simulink library "carnot"  (R2018b)
settings: Solver=VariableStepAuto  StartTime=0.0  StopTime=10.0  RelTol=1e-3
undefined symbols (not defined in the file or in its folder): A, A_earth, acol, Acol, ActPower1, ActPower2, ActPower3, Ad, Ad0, Ar, Au, Au0, Azimuth_Angle, B, Bd, Bd0, Br, Bu, Bu0, C, c1, c2, c3, c33, c4, c5, c6, CarnotCallbacks_Density, CarnotCallbacks_Enthalpy, CarnotCallbacks_Enthalpy2Temperature, CarnotCallbacks_Entropy, CarnotCallbacks_Evaporation_Enthalpy, CarnotCallbacks_GlobalMessageLevel, CarnotCallbacks_Grashof, CarnotCallbacks_Heat_Capacity, CarnotCallbacks_Kinematic_Viscosity, CarnotCallbacks_PMV_PPD, CarnotCallbacks_Prandtl, CarnotCallbacks_Saturation_Property, CarnotCallbacks_Saturation_Temperature, CarnotCallbacks_Saturation_Value_Water, CarnotCallbacks_Specific_Volume, CarnotCallbacks_Thermal_Conductivity, CarnotCallbacks_Vapour_Content, CarnotCallbacks_Vapour_Pressure, Cd, Cdl, Cr, Cu, Davies, Dd, DE_TRY2010_04_averageYear, delta_grd, density, DiameterLastPiece, dl, DPConstant, DPLinear, DPQuadratic, Dr ... (+59)
libraries: $bdroot x429, simulink x36, simulink_extras x12
(part 3 of 22)

== system carnot/Outputs ==
  AIV_selector : Subsystem  mask(AIV DATA){e1=on, e2=off, e3=off, e4=off, e5=off, e6=off, e7=off, e8=off, e9=off}
      mask prompts: e1 "Ts          : sensitive temperature, °C"; e2 "Tc          : convective/air temperature, °C"; e3 "Tr           : radiative temperature, °C"; e4 "x_H2O   : absolute water mass in air, kg/kg air"; e5 "x_CO2   : absolute CO2 mass in air, kg/kg air"; e6 "rho         : density of air, kg/m^3"; e7 "cp          : specific heat capacity of air, J/(kg*K)"; e8 "p            : absolute air pressure, N/m^2"; e9 "nair_out : air volume change indoors-outdoors, 1/h"
      mask help:
      | This block delivers a user specified vector with elements of the [AIV] vector.
      |
      | [AIV] : vector from NODE block
      | [AIV]s : output vector with user selected elements from [AIV]
      |
      | The sequence of elements in the output vector is identical to the sequence of selected check boxes counted from to the top to the bottom.
      mask init:
      | % concatenate elements of output "v":
      | v = [];
      | if (e1==1) v = [v 1]; end
      | if (e2==1) v = [v 2]; end
      | if (e3==1) v = [v 3]; end
      | if (e4==1) v = [v 4]; end
      | if (e5==1) v = [v 5]; end
      | if (e6==1) v = [v 6]; end
      | if (e7==1) v = [v 7]; end
      | if (e8==1) v = [v 8]; end
      | if (e9==1) v = [v 9]; end
      mask Help: web(fullfile(path_carnot('help'),'AIV_selector.html'),'-helpbrowser')
      mask Display:
      | plot ([0.8 0.9], [0.32 0.32])
      | plot ([0.8 0.85], [0.32 0.1])
      | plot ([0.9 0.85], [0.32 0.1])
      | plot ([0.827 0.827], [0 0.05])
      | plot ([0.827 0.87], [0.05 0.05])
      | plot ([0.87 0.87], [0 0.05])
      | plot ([0.827 0.87], [0 0])
  Display_THB1 : Subsystem  mask(display THB){t=on, m=off, p=off, id=off, mix=off, d=off}
      mask prompts: t "temperature [degree centigrade]"; m "massflow [kg/s]"; p "pressure [Pa]"; id "fluid ID (1 = water, 2 = air, 3 = cotton oil, 4 = water-glycol)"; mix "fluid mix"; d "diameter [m]"
      mask help: Displays the ticked values from one THB.
      mask init:
      | v=[];
      | if (t)
      |     v  = [2];
      | end
      | if (m)
      |     v= [v 3];
      | end
      | if (p)
      |     v = [v 4];
      | end
      | if (id)
      |     v = [v 5];
      | end
      | if (mix)
      |     v = [v 6];
      | end
      | if (d)
      |     v = [v 7];
      | end
      mask Help: web(fullfile(path_carnot('help'),'display_THB.html'),'-helpbrowser')
  Display_THB2 : Subsystem  mask(display THB){t=off, m=off, p=on, id=off, mix=off, d=off}
      mask prompts: t "temperature [degree centigrade]"; m "massflow [kg/s]"; p "pressure [Pa]"; id "fluid ID (1 = water, 2 = air, 3 = cotton oil, 4 = water-glycol)"; mix "fluid mix"; d "diameter [m]"
      mask help: Displays the ticked values from two THB.
      mask init:
      | v=[];
      | if (t)
      |     v  = [2];
      | end
      | if (m)
      |     v= [v 3];
      | end
      | if (p)
      |     v = [v 4];
      | end
      | if (id)
      |     v = [v 5];
      | end
      | if (mix)
      |     v = [v 6];
      | end
      | if (d)
      |     v = [v 7];
      | end
      mask Help: web(fullfile(path_carnot('help'),'display_THB.html'),'-helpbrowser')
  Display_THB3 : Subsystem  mask(display THB){t=off, m=off, p=on, id=off, mix=off, d=off}
      mask prompts: t "temperature [degree centigrade]"; m "massflow [kg/s]"; p "pressure [Pa]"; id "fluid ID (1 = water, 2 = air, 3 = cotton oil, 4 = water-glycol)"; mix "fluid mix"; d "diameter [m]"
      mask help: Displays the ticked values from four THB.
      mask init:
      | v=[];
      | if (t)
      |     v  = [2];
      | end
      | if (m)
      |     v= [v 3];
      | end
      | if (p)
      |     v = [v 4];
      | end
      | if (id)
      |     v = [v 5];
      | end
      | if (mix)
      |     v = [v 6];
      | end
      | if (d)
      |     v = [v 7];
      | end
      mask Help: web(fullfile(path_carnot('help'),'display_THB.html'),'-helpbrowser')
  Display_THB4 : Subsystem  mask(display THB){t=on, m=off, p=off, id=off, mix=off, d=off}
      mask prompts: t "temperature [degree centigrade]"; m "massflow [kg/s]"; p "pressure [Pa]"; id "fluid ID (1 = water, 2 = air, 3 = cotton oil, 4 = water-glycol)"; mix "fluid mix"; d "diameter [m]"
      mask help: Displays the ticked values from four THB
      mask init:
      | v=[];
      | if (t)
      |     v  = [2];
      | end
      | if (m)
      |     v= [v 3];
      | end
      | if (p)
      |     v = [v 4];
      | end
      | if (id)
      |     v = [v 5];
      | end
      | if (mix)
      |     v = [v 6];
      | end
      | if (d)
      |     v = [v 7];
      | end
      mask Help: web(fullfile(path_carnot('help'),'display_THB.html'),'-helpbrowser')
  Display_THB5 : Subsystem  mask(display THB){t=on, m=off, p=off, id=off, mix=off, d=off}
      mask prompts: t "temperature  [degree centigrade]"; m "massflow [kg/s]"; p "pressure [Pa]"; id "fluid ID (1 = water, 2 = air, 3 = cotton oil, 4 = water-glycol)"; mix "fluid mix"; d "diameter [m]"
      mask help: Displays the ticked values from six THB.
      mask init:
      | v=[];
      | if (t)
      |     v  = [2];
      | end
      | if (m)
      |     v= [v 3];
      | end
      | if (p)
      |     v = [v 4];
      | end
      | if (id)
      |     v = [v 5];
      | end
      | if (mix)
      |     v = [v 6];
      | end
      | if (d)
      |     v = [v 7];
      | end
      mask Help: web(fullfile(path_carnot('help'),'display_THB.html'),'-helpbrowser')
  Display_THB6 : Subsystem  mask(display THB){t=on, m=off, p=off, id=off, mix=off, d=off}
      mask prompts: t "temperature  [degree centigrade]"; m "massflow [kg/s]"; p "pressure [Pa]"; id "fluid ID (1 = water, 2 = air, 3 = cotton oil, 4 = water-glycol)"; mix "fluid mix"; d "diameter [m]"
      mask help: Displays the ticked values from six THB.
      mask init:
      | v=[];
      | if (t)
      |     v  = [2];
      | end
      | if (m)
      |     v= [v 3];
      | end
      | if (p)
      |     v = [v 4];
      | end
      | if (id)
      |     v = [v 5];
      | end
      | if (mix)
      |     v = [v 6];
      | end
      | if (d)
      |     v = [v 7];
      | end
      mask Help: web(fullfile(path_carnot('help'),'display_THB.html'),'-helpbrowser')
  PMV_PPD : Subsystem  LoadFcn=CarnotCallbacks_PMV_PPD('LoadFcn', gcb);  mask(PMV_PPD){DEBUGLEVEL=WARNINGLEVEL, MAXTOTALWARNINGS=inf, MAXCONSECUTIVEWARNINGS=inf, WRITETOFILE=0, FILENAME='messages.txt'}
      mask prompts: DEBUGLEVEL "Debug level"; MAXTOTALWARNINGS "maximum number of total warning"; MAXCONSECUTIVEWARNINGS "maximum number of consecutive warnings"; WRITETOFILE "write messages to file"; FILENAME "filename for messages"
      mask help:
      | This block calculates from it's inputs the thermal comfort according to PMV (pedicted mean vote) and PPD (predicted percentage of dissatisfied).
      | LoadPerPerson : metabolic rate of persons per surface in W/m² (typical 58.2 W/m²)
      | MechanicalLoad : effective mechanical power of a person in W/m²
      | ClothingIsolation : thermal resistance of the clothing in [m²/kW]; 1 clo = 0.155 W/m²
      | air temperature [°C]
      | radiation temperature [°C]
      | relative air velocity [m/s]
      | PartialPressureVapur : partial pressure of water [Pa]
      mask init:
      | %global debug level
      | [DEBUGLEVEL, MAXTOTALWARNINGS, MAXCONSECUTIVEWARNINGS, WRITETOFILE, FILENAME] = CarnotCallbacks_PMV_PPD('CheckDebugLevels', DEBUGLEVEL, MAXTOTALWARNINGS, MAXCONSECUTIVEWARNINGS, WRITETOFILE, FILENAME);
      mask Help: web(fullfile(path_carnot('help'),'PMV_PPD.html'),'-helpbrowser')
      mask TypeOptions DEBUGLEVEL: DEBUGLEVEL | INFOLEVEL | WARNINGLEVEL | ERRORLEVEL | FATALLEVEL | NOLEVEL
      mask Callback DEBUGLEVEL: CarnotCallbacks_PMV_PPD('MaskVisibilities');
      mask DialogControl ParameterTabVar0 Prompt: debugging air property calculations
  S_selector : Subsystem  mask(S_Selector){e1=on, e2=off, e3=off, e4=off, e5=off, e6=off, e7=off, e8=off, e9=off, e10=off, e11=off, e12=off, e13=off}
      mask prompts: e1 "Qdot_sol       : solar radition load, W"; e2 "Qdot_equip   : electric equipment load, W"; e3 "Qdot_light     : electric light load, W"; e4 "Qdot_pers     : person load, W"; e5 "Qdot_heat     : heating / cooling, W"; e6 "Qdot_air        : heating/cooling power of air change, W"; e7 "Qdot_c          : heat flow to convective node, W"; e8 "Qdot_r           : heat flow to radiative node, W"; e9 "mdot_air        : air mass flow, kg/s"; e10 "mdot_H2O    : water mass flow, kg/s"; e11 "mdot_CO2    : CO2 mass flow, kg/s"; e12 "Vdot_out2in  : air volume flow outdoors -> indoors, m^3/s"; e13 "Vdot_in2out  : air volume flow indoors -> outdoors, m^3/s"
      mask help:
      | This block delivers a user specified vector with elements of the [S] vector.
      |
      | [S] : vector from SOURCE or SINK block
      | [S]s : output vector with user selected elements from [S]
      |
      | The sequence of elements in the output vector is identical to the sequence of selected check boxes counted from to the top to the bottom.
      mask init:
      | % concatenate elements of output "v":
      | v = [];
      | if (e1==1) v = [v 1]; end
      | if (e2==1) v = [v 2]; end
      | if (e3==1) v = [v 3]; end
      | if (e4==1) v = [v 4]; end
      | if (e5==1) v = [v 5]; end
      | if (e6==1) v = [v 6]; end
      | if (e7==1) v = [v 7]; end
      | if (e8==1) v = [v 8]; end
      | if (e9==1) v = [v 9]; end
      | if (e10==1) v = [v 10]; end
      | if (e11==1) v = [v 11]; end
      | if (e12==1) v = [v 12]; end
      | if (e13==1) v = [v 13]; end
      mask Help: web(fullfile(path_carnot('help'),'S_selector.html'),'-helpbrowser')
      mask Display:
      | plot ([0.8 0.9], [0.32 0.32])
      | plot ([0.8 0.85], [0.32 0.1])
      | plot ([0.9 0.85], [0.32 0.1])
      | plot ([0.827 0.827], [0 0.05])
      | plot ([0.827 0.87], [0.05 0.05])
      | plot ([0.87 0.87], [0 0.05])
      | plot ([0.827 0.87], [0 0])
  Sensitive_Room_Temperature : Subsystem  mask(SENSITIVE TEMPERATURE){share_c=47}
      mask prompts: share_c "SHARE of convective sensitivity, [0,100%]:"
      mask help:
      | This block merges the convective and radiative zone node temperature to the SENSITIVE ZONE TEMPERATURE (weighted arithmetic average of both components).
      | [T] = [Tc; Tr]:  temperature vector of node, °C
      | Ts:              sensitive zone temperature, °C
      mask init:
      | blockname = gcb;
      | 
      | if (length(share_c)~=1) error(['PARAMETERS block "' blockname ': "SHARE of ..." must have only 1 entry !']); end;
      | if (share_c<0) | (share_c>100) error(['PARAMETERS block "' blockname '" : "SHARE of ..." must be within [0, 100%] !']); end;
      | share_c = share_c/100;
      mask Help: web(fullfile(path_carnot('help'),'Sensitive_room_temperature.html'),'-helpbrowser')
  THV_select : Subsystem  mask(select from THV){f=off, t=on, m=off, p=off, id=off, mix=off, d=off, dpcon=off, dplin=off, dpqua=off}
      mask prompts: f "flow identifier"; t "temperature [degree centigrade]"; m "massflow [kg/s]"; p "pressure [Pa]"; id "fluid ID (1 = water, 2 = air, 3 = cotton oil, 4 = water-glycol)"; mix "fluid mix"; d "diameter [m]"; dpcon "constant press. drop"; dplin "linear pressure drop"; dpqua "quadratic pressure drop"
      mask help: Selects the ticked values from the thermo hydraulic vector.
      mask init:
      | v=[];
      | if (f)
      |     v  = [1];
      | end
      | if (t)
      |     v  = [v 2];
      | end
      | if (m)
      |     v= [v 3];
      | end
      | if (p)
      |     v = [v 4];
      | end
      | if (id)
      |     v = [v 5];
      | end
      | if (mix)
      |     v = [v 6];
      | end
      | if (d)
      |     v = [v 7];
      | end
      | if (dpcon)
      |     v = [v 8];
      | end
      | if (dplin)
      |     v = [v 9];
      | end
      | if (dpqua)
      |     v = [v 10];
      | end
      mask Help: eval('man(''THV_select'')')
  display_weather : Subsystem  mask(Select weather data){pos=off, sun_beam=off, sun_dfu=off, rad=on, ta=off, ts=off, pre=off, rh=off, ci=off, p=off, ws=off, wd=off, col=off}
      mask prompts: pos "sunposition [zenith azimuth incidence] angles [degree]"; sun_beam "solar beam radiation on a normal surface [W/m²]"; sun_dfu "solar diffuse radiation on a horizontal surface [W/m²]"; rad "solar radiation on the surface [direct diffuse] [W/m²]"; ta "ambient temperature [degree centigrade]"; ts "sky temperature [degree centigrade]"; pre "precipitation [m/s]"; rh "relative humidity [percent]"; ci "cloud index [0=no cloud 1= covered]"; p "pressure [Pa]"; ws "wind speed [m/s]"; wd "wind direction (0°=north 270°=east) [degree]"; col "collector [incidence parallel_incidence perpendicular] [degree]"
      mask help: Selects the ticked weather data from the input weather data vector.
      mask init:
      | v=[];
      | if (pos)
      |     v  = [2 3 14];
      | end
      | if (sun_beam)
      |     v= [v 4];
      | end
      | if (sun_dfu)
      |     v= [v 5];
      | end
      | if (rad)
      |     v= [v 17 18];
      | end
      | if (ta)
      |     v = [v 6];
      | end
      | if (ts)
      |     v = [v 7];
      | end
      | if (rh)
      |     v = [v 8];
      | end
      | if (pre)
      |     v = [v 9];
      | end
      | if (ci)
      |     v = [v 10];
      | end
      | if (p)
      |     v = [v 11];
      | end
      | if (ws)
      |     v = [v 12];
      | end
      | if (wd)
      |     v = [v 13];
      | end
      | if (col)
      |     v = [v 14 15 16];
      | end
      mask Help: web(fullfile(path_carnot('help'),'display_weather.html'),'-helpbrowser')
  printer : S-Function  FunctionName=printer  SFunctionDeploymentMode=off  EnableBusSupport=off  mask(printer){}
      mask help: Print the input to the MATLAB command window during iterations of SIMULINK
      mask Help: web(fullfile(path_carnot('help'),'printer.html'),'-helpbrowser')

== system carnot/Source ==
  Boiler : Subsystem
      mask Display: plot(-20,0,120,100,[10,90,90,10,10],[10,10,20,20,10],[80,80,20,20],[20,90,90,20],[20,70,70,20],[24,24,30,30],[32,30,28],[30,40,30],[43,40,38],[30,40,30],[53,50,47],[30,40,30],[63,60,57],[30,40,30],[35,32,30,29,31,36,39,40,37,35],[75,69,65,58,50,49,53,59,68,75],[57,54,51,51,53,58,62,62,59,57],[76,71,67,58,49,48,54,60,69,76])
  Chiller : Subsystem
      mask Display: plot(20,20,80,100,(100-[30,46,36,46,36,46,30]),[40,40,50,60,70,80,80],(100-[70,54,64,54,64,54,64,54,64,54,70]),[40,40,44,50,55,60,65,70,75,80,80],[56,45],[95,95],[51,51],[82,95])
  Cogeneration : Subsystem
      mask Display: plot(0.1, 0, 0.9, 1,([0,8,20,30,42,50,50,42,30,20,8,0,0]+20)/140, [60,74,80,80,74,60,40,27,20,20,27,40,60]/100,([40,40,25,10,10]+20)/140,[40,60,50,60,40]/100,[60,50]/100,[50,50]/100,[60,80,80,60,60]/100, [30,30,70,70,30]/100,([90,97,97,90,80,75,75,80,90,97]+12)/140, [50,50,40,35,35,40,60,65,65,60]/100)
  Electric_Generator : Subsystem
      mask Display: plot(0,0,100,100,[40,20],[50,50],[40,40],[30,70],[50,50],[-0,100],[70,50],[50,50])
  Energy : Subsystem
      mask Display: plot(0,-0.1,0.8,1,[90,67,84,63,80,60,70,90,80,80,70,20,10,10,20,60]/120,[70,87,64,83,60,80,90,70,60,10,0,0,10,70,80,80]/100,[30,60,60,40,40,50,50,40,40,30,30]/120,[60,60,50,50,40,40,30,30,10,10,60]/100)
  Heat_Exchanger : Subsystem
      mask Display: plot(0,0,100,100,[70,30,30,70,70,30],[90,10,90,90,10,10])
  Heat_Pump : Subsystem
      mask Display: plot(20,20,80,100,[30,46,36,46,36,46,30],[40,40,50,60,70,80,80],[70,54,64,54,64,54,64,54,64,54,70],[40,40,44,50,55,60,65,70,75,80,80],[56,45],[95,95],[51,51],[82,95])
  Simple : Subsystem
      mask Display: plot(0,0,100,100,[30,40,60,70,70,30,30],[50,44,44,50,10,10,50],[50,50],[44,57],[50,46,44,46,50,54,56,54,50],[93,85,70,54,48,54,70,85,93])
  Solar_Thermal : Subsystem
      mask Display: plot(0,0,100,100,[0,10,16,19,20],[80,81,84,90,100],[7,10],[79,60],[17,30],[84,70],[21,40],[94,90],[30,90,100,40,30],[10,70,60,-0,10],[90,90,40,33],[70,60,10,13],[89,39],[61,12])
  Ventilation : Subsystem
      mask Display:
      | plot([0.2 0.35], [0.8 0.7])
      | plot([0.35 0.65], [0.7 0.7])
      | plot([0.65 0.8], [0.7 0.8])
      | plot([0.65 0.8], [0.76 0.8])
      | plot([0.7 0.8], [0.65 0.8])
      | plot([0.2 0.35], [0.2 0.3])
      | plot([0.35 0.65], [0.3 0.3])
      | plot([0.65 0.8], [0.3 0.2])
      | plot([0.2 0.25], [0.2 0.32])
      | plot([0.2 0.35], [0.2 0.23])
      | plot ([0.45 0.45], [0 1])
      | plot ([0.55 0.55], [0 1])
      | plot ([0.45 0.55], [0.2 0.2])
      | plot ([0.45 0.55], [0.8 0.8])
      | plot ([0.45 0.55], [0 0.2])
      | plot ([0.45 0.55], [0.8 1])

== system carnot/Storage ==
  Electric : Subsystem
      mask Display: plot(0,-10,100,100,[70,70,60,40,30,30,40,60,70,60,40,30],[80,10,-0,-0,10,80,70,70,80,90,90,80],[44,47,54,57,54,47,44],[80,76,76,80,84,84,80])
  Thermal : Subsystem
      mask Display: plot(30,40,60,90,[36,36,40,50,54,54,50,40,36],[90,50,45,45,50,90,93,93,90],[36,51,40,51,36],[74,74,79,85,85],[36,51,44,51,36],[54,54,56,58,58])

== system carnot/Toolbox ==
  Average : Subsystem  mask{time_intervall=3600, offset_flag=off, enable_flag=off}
      mask prompts: time_intervall "Delta_t in s"; offset_flag "start calculating every full hour"; enable_flag "only calculate when enabled"
      mask help:
      | This block calculates the average of each input vector during a specified time Delta_t. During this time interval the output is held.
      | The output time is the time of the last average calculation. Every time the average is calculated again, a signal pulse of 1 is put out.
      | When the full hour flag is set, the calculation of the average is started every full hour once again.
      | When the enable flag is set, the functions calculates only while the enable signal is 1. When it is 0, the function repeats putting out the last output.
      mask init:
      | if time_intervall==0
      |     delta_t = 1;
      | else
      |     delta_t = time_intervall;
      | end
      mask Help: web(fullfile(path_carnot('help'),'Average.html'),'-helpbrowser')
  Count_Working_Time : S-Function  FunctionName=countcycles  SFunctionDeploymentMode=off  EnableBusSupport=off  mask(count working time){}
      mask help: This block counts the number of on cycles and the working time (time when input is above zero).
      mask Help: web(fullfile(path_carnot('help'),'Count_Working_Time.html'),'-helpbrowser')
      mask Display:
      | port_label('input', 1, 'Input')
      | port_label('output', 1, 'flank')
      | port_label('output', 2, 'cycles')
      | port_label('output', 3, 'actual worktime')
      | port_label('output', 4, 'total worktime')
  Date2Sec : S-Function  FunctionName=date2sec_s  SFunctionDeploymentMode=off  EnableBusSupport=off
      mask help:
      | This function calculates for a given date the sum of seconds in the year.
      | The input Year is a dummy argument.
      | 0 s is january, 1st at 0:00:00.
      |
      | INPUT VECTOR:
      | date [year month day hour minute second]
      |
      | OUTPUT VECTOR:
      | date [s]
  Economy_Ecology : Subsystem  mask(economy_ecology){}
      mask help: Calculates massflow, costs, exhaust gas etc.
      mask Help: web(fullfile(path_carnot('help'),'economy_ecology.html'),'-helpbrowser')
  GlobalMessageLevel : Subsystem  LoadFcn=CarnotCallbacks_GlobalMessageLevel('LoadFcn');  mask(Global Message Level){GLOBALLOCAL=local, DEBUGLEVEL=DEBUG, MAXTOTALWARNINGS=inf, MAXCONSECUTIVEWARNINGS=inf, WRITETOFILE=0, FILENAME='error.txt'}
      mask prompts: GLOBALLOCAL "message settings"; DEBUGLEVEL "message level"; MAXTOTALWARNINGS "maximum total number of warnings"; MAXCONSECUTIVEWARNINGS "maxmum consecutive warnings"; WRITETOFILE "write messages to file"
      mask help:
      | This block sets the message level of the complete model. Error messages and warnings are generated for example by the material properties functions (density, ...), see library Basic/Material_Properties for the blocks.
      | local - settings are defined by each block individually
      | global - settings are defined by this GlobalMessageLevel block
      | Copy this block once in the model if you want to use a global handling of Carnot error messages.
      mask init:
      | CarnotCallbacks_GlobalMessageLevel('SetData');
      mask TypeOptions GLOBALLOCAL: global | local
      mask Callback GLOBALLOCAL: CarnotCallbacks_GlobalMessageLevel('MaskCallback');
      mask TypeOptions DEBUGLEVEL: DEBUGLEVEL | INFOLEVEL | WARNINGLEVEL | ERRORLEVEL | FATALLEVEL | NOLEVEL
      mask Display:
      | fprintf(get_param(gcb, 'GLOBALLOCAL'));
      | fprintf(['\n\n', get_param(gcb, 'DEBUGLEVEL')]);
  ModelDoc : Subsystem  mask(ModelDoc){}
      mask init:
      | % modelname=bdroot;
      | % filename=[modelname '_params.txt'];
      | % fid = fopen(filename, 'w');
      | % line='______________________________________________________';
      | % ttt=SearchWriteParams(modelname,fid);
      | % fclose(fid);
      | 
      | ok = CarnotCallbacks_ModelDoc;
      settings: OpenFcn=|
      | if  ~BlockIsInCarnotLibrary
      |     modelname=get_param(0,'CurrentSystem');
      |     filename=[modelname '_params.txt'];
      |     open(filename);
      | end
      mask Display: disp('Model Description\n Update Model <Ctrl>D \n before double-clicking');
  RealDate : Subsystem  mask{form=second}
      mask prompts: form "Selector"
      mask help:
      | This functions puts out the system time and date:
      | Year - current year
      | Month - current month
      | Day - current day in the month (date)
      | Hour -  current hour (time)
      | Minute - current minute (of the time)
      | Second - current second (of the time)
      mask Help: web(fullfile(path_carnot('help'),'RealDate.html'),'-helpbrowser')
      mask TypeOptions form: year | month | day | hour | minute | second
  RealTime : Subsystem
      mask help:
      | This functions puts out the system time in seconds.
      | Output 0 s means January, 1st 0:00
      mask Help: web(fullfile(path_carnot('help'),'RealTime.html'),'-helpbrowser')
  RealTimePulse : Subsystem  mask{typ=rising, time=3}
      mask prompts: typ "type"; time "time interval [s]"
      mask help:
      | This functions creates a signal pulse, whenever the input pulse is
      | changing as specified. The duration of the pulse is depending on the system time, not the simulation time.
      |
      | INPUT VECTOR:
      |   in : signal to start pulse [0,1]
      |
      | OUTPUT VECTOR:
      |  out : new pulse [0,1]
      mask Help: web(fullfile(path_carnot('help'),'RealTimePulse.html'),'-helpbrowser')
      mask TypeOptions typ: rising | falling | either
  Sec2Date : S-Function  FunctionName=sec2date_s  SFunctionDeploymentMode=off  EnableBusSupport=off
      mask help:
      | This functions calculates from a given number of seconds the date.
      |
      | INPUT VECTOR:
      | - time [s]
      |
      | OUTPUT VECTOR:
      | - date [month day hour minute second]
  SumTime : S-Function  FunctionName=sumtime_s  SFunctionDeploymentMode=off  EnableBusSupport=off
      mask help:
      | This function calcultes for a given date the sum of seconds, minutes, ... in the year.
      |
      | INPUT VECTOR:
      | date [year month day hour minute second]
      |
      | OUTPUT VECTOR:
      | sum of |year month day hour minute second]
      mask Help: web(fullfile(path_carnot('help'),'SumTime_mdl.html'),'-helpbrowser')
      mask Display: plot(0,0,70,60,[40 20 35 20 40],[50 50 30 10 10],[50 50 45 55 50  50 52 54],[45 35 35 35 35 20 17 15]);
  SystemPulse : Subsystem  mask(system pulse){enable_flag=on, datecheck=off, date=[2 10 10 36 15], period=5, pulsewidth=2}
      mask prompts: enable_flag "Wait for enabling pulse"; datecheck "Wait for start date"; date "start date [month day hour minute second]"; period "period [s]"; pulsewidth "pulse width [s]"
      mask help:
      | This block generates a discrete pulse of 0 and 1, but this pulse depends on the system time, not the simulation time.
      | If the date flag is set, the function starts pulsing only when the system date reaches the specified date. Otherwise the output is 0.
      | If the enable flag is set, the function waits, until the enabling pulse once rise from 0 to 1. Afterwards the pulsing is started. Before pulsing the output will be 0.
      mask Help: web(fullfile(path_carnot('help'),'SystemPulse.html'),'-helpbrowser')
  THB2THV : Subsystem  InitFcn=load('THB.mat');  mask(THB2THV){}
      mask help: This block converts the Thermo-Hydraulic-Bus to the old Thermo-Hydraulic-Vector.
      mask Help: web(fullfile(path_carnot('help'),'THB2THV.html'),'-helpbrowser')
  THBMemory : Subsystem  InitFcn=load('THB.mat');  mask(THB Memory){ID=20001, T=20, mdot=0, p=1e5, FluidType=1, FluidMix=0, d=0.01, c=0, l=0, q=0, LH=1000, H=0, Annotation_ID=off, Annotation_T=off, Annotation_mdot=off, Annotation_p=off, Annotation_FluidType=off, Annotation_FluidMix=off, Annotation_d=off, Annotation_c=off, Annotation_l=off, Annotation_q=off, Annotation_LH=off, Annotation_H=off}
      mask prompts: ID "Fluid ID [1]"; T "Temperature [°C]"; mdot "Mass flow rate [kg/s]"; p "Pressure [Pa]"; FluidType "Fluid type [enum]"; FluidMix "Fluid mix [1]"; d "Diameter of the last piece [m]"; c "Constant pressure drop coefficient [Pa]"; l "Linear pressure drop coefficient [Pa/(kg/s)]"; q "Quadratic pressure drop coefficient [Pa/(kg/s)²]"; LH "Hydraulic inductance [1/m]"; H "Geodetic height [m]"; Annotation_ID "Fluid ID as annotation"; Annotation_T "Temperature as annoation"; Annotation_mdot "Mass flow rate as annoation"; Annotation_p "Pressure as annotation"; Annotation_FluidType "Fluid type as annotation"; Annotation_FluidMix "Fluid mix as annotation"; Annotation_d "Diameter of the last piece as annotation"; Annotation_c "Constant pressure drop coefficient as annotation"; Annotation_l "Linear pressure drop coefficient as annotation"; Annotation_q "Quadratic pressure drop coefficient as annotation"; Annotation_LH "Hydraulic inductance as annotation"; Annotation_H "Geodetic height as annotation"
      mask help: This is a memory block for a complete THB.
      mask init:
      | %annotations    
      | MaskValues=get_param(gcb,'MaskValues');
      | AnnotationString='';
      | if strcmp(MaskValues{13},'on') %ID
      |     if ~isempty(AnnotationString)
      |         AnnotationString=[AnnotationString,sprintf('\n')];
      |     end
      |     AnnotationString=[AnnotationString,'ID ',MaskValues{1}];
      | end
      |     
      | if strcmp(MaskValues{14},'on') %T
      |     if ~isempty(AnnotationString)
      |         AnnotationString=[AnnotationString,sprintf('\n')];
      |     end
      |     AnnotationString=[AnnotationString,MaskValues{2}, ' °C temperature'];
      | end
      |     
      | if strcmp(MaskValues{15},'on') %T
      |     if ~isempty(AnnotationString)
      |         AnnotationString=[AnnotationString,sprintf('\n')];
      |     end
      |     AnnotationString=[AnnotationString,MaskValues{3}, ' kg/s mass flow rate'];
      | end
      |     
      | if strcmp(MaskValues{16},'on') %p
      |     if ~isempty(AnnotationString)
      |         AnnotationString=[AnnotationString,sprintf('\n')];
      |     end
      |     AnnotationString=[AnnotationString,MaskValues{4}, ' Pa pressure'];
      | end
      | 
      | if strcmp(MaskValues{17},'on') %type
      |     if ~isempty(AnnotationString)
      |         AnnotationString=[AnnotationString,sprintf('\n')];
      |     end
      |     AnnotationString=[AnnotationString,'fluid type ',MaskValues{5}];
      | end
      |     
      | if strcmp(MaskValues{18},'on') %mix
      |     if ~isempty(AnnotationString)
      |         AnnotationString=[AnnotationString,sprintf('\n')];
      |     end
      |     AnnotationString=[AnnotationString,MaskValues{6}, ' fluid mix'];
      | end
      |     
      | if strcmp(MaskValues{19},'on') %d
      |     if ~isempty(AnnotationString)
      |         AnnotationString=[AnnotationString,sprintf('\n')];
      |     end
      |     AnnotationString=[AnnotationString,MaskValues{7}, ' m diameter last piece'];
      | end
      |     
      | if strcmp(MaskValues{20},'on') %c
      |     if ~isempty(AnnotationString)
      |         AnnotationString=[AnnotationString,sprintf('\n')];
      |     end
      |     AnnotationString=[AnnotationString,MaskValues{8}, ' Pa constant pressure loss coefficient'];
      | end
      |     
      | if strcmp(MaskValues{21},'on') %l
      |     if ~isempty(AnnotationString)
      |         AnnotationString=[AnnotationString,sprintf('\n')];
      |     end
      |     AnnotationString=[AnnotationString,MaskValues{9}, ' Pa/(kg/s) linear pressure loss coefficient'];
      | end
      |     
      | if strcmp(MaskValues{22},'on') %q
      |     if ~isempty(AnnotationString)
      |         AnnotationString=[AnnotationString,sprintf('\n')];
      |     end
      |     AnnotationString=[AnnotationString,MaskValues{10}, ' Pa/(kg/s)² quadratic pressure loss coefficient'];
      | end
      |     
      | if strcmp(MaskValues{23},'on') %LH
      |     if ~isempty(AnnotationString)
      |         AnnotationString=[AnnotationString,sprintf('\n')];
      |     end
      |     AnnotationString=[AnnotationString,MaskValues{11}, ' 1/m hydraulic inductance'];
      | end
      |     
      | if strcmp(MaskValues{24},'on') %H
      |     if ~isempty(AnnotationString)
      |         AnnotationString=[AnnotationString,sprintf('\n')];
      |     end
      |     AnnotationString=[AnnotationString,MaskValues{12}, ' m geodetic height'];
      | end
      |     
      | set_param(gcb,'AttributesFormatString',AnnotationString);
      | 
      | clear MaskValues AnnotationString;
      mask Help: web(fullfile(path_carnot('help'),'THBMemory.html'),'-helpbrowser')
      mask DialogControl ParameterTabVar0 Prompt: values
      mask DialogControl ParameterTabVar01 Prompt: annotations
  THV2THB : Subsystem  InitFcn=load('THB.mat');  mask(THV2THB){}
      mask help: This block converts the old Thermo-Hydraulic-Vector to the Thermo-Hydraulic-Bus.
      mask Help: web(fullfile(path_carnot('help'),'THV2THB.html'),'-helpbrowser')
  UnitConv : Subsystem  mask{input_unit='kW/(m*h)', output_unit='W/(cm*min)'}
      mask prompts: input_unit "input unit"; output_unit "output unit"
      mask help:
      | This function converts the input from a specified unit to another specified unit.
      |   When specifying a unit, the unit symbols have to be separated by * or /.
      |   That means kWh has to be written as kW*h.
      |
      | !!! Use of this block on your own risk. This block converts not all units correctly !!!
      |
      | INPUT VECTOR
      |   in : value of input unit
      |
      | OUTPUT VECTOR
      |   out : input value converted to value of output unit
      mask Help: web(fullfile(path_carnot('help'),'UnitConv.html'),'-helpbrowser')
  UnitConv_Temperature : Subsystem  mask(temperature unit conversion){ini_unit=°C, fin_unit=°F}
      mask prompts: ini_unit "initial unit of the temperature"; fin_unit "target unit of the temperature"
      mask help:
      | converts a temperature form a unit to another.
      |
      | initial unit and target unit should be one of the following characters :
      |   - '°C' : Celsius
      |   - 'K' : Kelvin
      |   - '°F' : Farenheit
      |
      | Warning : a difference of temperature doesn't need to be convert from
      | Kelvin to Celsius.
      mask Help: web(fullfile(path_carnot('help'),'UnitConv_Temperature_mdl.html'),'-helpbrowser')
      mask TypeOptions ini_unit: °C | K | °F
      mask TypeOptions fin_unit: °C | K | °F
  WDB2Weather : Subsystem  mask(WDB 2 weather){}
      mask help:
      | Creates the weather data vector from the weather data bus WDB.
      | Format in weather data vector:
      | 1  timevalue (comment line) format YYYYMMDDHHMM    -
      | 2  zenith angle of sun (at time, not averaged)       degree
      | 3  azimuth angle of sun (0°=south, east negative) degree
      | 4  beam solar radiation on a normal surface         W/m^2
      | 5  diffuse solar radiation on a horizontal surface   W/m^2
      | 6  ambient temperature                                    degree celsius
      | 7  radiation temperature of sky                          degree celsius
      | 8  relative humidity                                           percent
      | 9  precipitation                                                 m/s
      | 10 cloud index (0=no cloud, 1=covered sky)         -
      | 11 station pressure                                           Pa
      | 12 mean wind speed                                         m/s
      | 13 wind direction (north=0° west=270°)             degree
      | 14 incidence angle on surface (0° = vertical)      degree
      | 15 longitudinal incidence angle                       degree
      | 16 transversal incidence angle                        degree
      | 17 direct solar radiation on surface                 W/m²
      | 18 diffuse solar radiation on surface                W/m²
  Wait : Subsystem  mask{check=off, date=[1 10 15 31 00], wtime=1}
      mask prompts: check "Look for start date"; date "start date [month day hour minute second]"; wtime "waiting time [s]"
      mask help:
      | This function waits until the system time reaches the given date.
      | Whenever called again, this function will wait for the given number of seconds.
      mask init:
      | if check==0
      |  date(1) = -1;
      | end;
      mask Help: web(fullfile(path_carnot('help'),'Wait.html'),'-helpbrowser')
      mask Display: plot(-31,-31,31,31,[0     9    17    23    28    30    29    26    20    13     4    -5 -13   -21   -26   -29   -30   -28   -23   -17    -8 1],[ 30    29    25    19    11     2    -7   -15   -22   -27   -30   -30 -27   -22   -15    -6     3    11    19    25    29 30],[-20,0,0],[0,0,20])
  Weather2WDB : Subsystem  mask(weather 2 WDB){}
      mask help:
      | Creates the weather data bus WDB from the weather data vector.
      | Format in weather data vector:
      | 1  timevalue (comment line) format YYYYMMDDHHMM    -
      | 2  zenith angle of sun (at time, not averaged)       degree
      | 3  azimuth angle of sun (0°=south, east negative) degree
      | 4  beam solar radiation on a normal surface         W/m^2
      | 5  diffuse solar radiation on a horizontal surface   W/m^2
      | 6  ambient temperature                                    degree celsius
      | 7  radiation temperature of sky                          degree celsius
      | 8  relative humidity                                           percent
      | 9  precipitation                                                 m/s
      | 10 cloud index (0=no cloud, 1=covered sky)         -
      | 11 station pressure                                           Pa
      | 12 mean wind speed                                         m/s
      | 13 wind direction (north=0° west=270°)             degree
      | 14 incidence angle on surface (0° = vertical)      degree
      | 15 longitudinal incidence angle                       degree
      | 16 transversal incidence angle                        degree
      | 17 direct solar radiation on surface                 W/m²
      | 18 diffuse solar radiation on surface                W/m²
  write_txt_file : Subsystem  mask{clear=off, filename='testout.txt'}
      mask prompts: clear "clear existing file"
      mask help:
      | This function writes the input data to a ascii-txt-file, so it can be opened with an usual editor.
      | The data is only written, when the enable signal is 1.
      | It's possible to append data to an existing file or to clear the file before writing.
      |
      | INPUT VECTOR
      |   in         : input data
      |   enable : signal [0,1]
      mask Help: web(fullfile(path_carnot('help'),'write_txt_file.html'),'-helpbrowser')

== system carnot/Weather ==
  Add_Solar_Position : Subsystem  mask(sun position){longi=-7, lati=50, timezone=-15}
      mask prompts: longi "geographical longitude [degrees] (east negative)"; lati "geographical latitude [degrees] (north positive)"; timezone "longitude of timezone [degrees] (east negative)"
      mask help:
      | This funktion calculates the sun position  and sets it in the weather data vector. Solar zenith angle and azimuth angle (in degrees) (east negative, south = 0°) are set in the weather vector.
      | Timezones:    GMT = 0
      |                       MEZ = -15
      |                       MESZ = -30
      mask init:
      | longi = min(180, max(-180, longi));
      | lati = min(90, max(-90, lati));
      | timezone = min(360, max(-360, timezone));
      mask Help: web(fullfile(path_carnot('help'),'Solar_Position.html'),'-helpbrowser')
  DWD_TRY_Radiation_Filter : Subsystem  mask(DWD TRY Filter){f=5}
      mask prompts: f "Filter llevel (1 = high, 10 = low)"
      mask help:
      | Filter for solar beam radiation of test reference years 2010 of the german DWD.
      | The original data has some defaults which results in a wrong time-vector (and solar position).
      mask Help: web(fullfile(path_carnot('help'),'DWD_TRY_Radiation_Filter.html'),'-helpbrowser')
  Fixed_Surface : Subsystem  mask(fixed surface){colangle=0, colazi=0, colrot=0}
      mask prompts: colangle "Slope of surface (0° = horizontal) [degree]"; colazi "Azimuth of surface (0° = south, -90° = east) [degree]"; colrot "Rotation angle of surface [degree]"
      mask help:
      | Set collector or surface to a fixed position.
      | All angles are limited to the range -180 ° ... +180 °
      mask init:
      | colangle = min(180, max(-180, colangle));
      | colazi = min(180, max(-180, colazi));
      | colrot = min(180, max(-180, colrot));
      mask Help: web(fullfile(path_carnot('help'),'Fixed_Surface.html'),'-helpbrowser')
      mask Display:
      | disp(['Inclination: ' get_param(gcb,'colangle') '°\n\n'])
      | disp(['\n\nAzimuth   : ' get_param(gcb,'colazi') '°\n\n'])
      | disp(['\n\nRotation  : ' get_param(gcb,'colrot') '°'])
  Radiation_on_Inclined_Surface : Subsystem  mask(inclined surface){sky=Perez 1990, reflect=0.2}
      mask prompts: sky "sky model"; reflect "ground reflectance (0..1)"
      mask help: Calculates the radiation on inclined surfaces from sun-position (zenith angle and azimuth). The radiation and incidence angles for the inclined surface are set in the weather vector. All angles are in degrees.
      mask init:
      | reflect = min(1.0, max(0.0, reflect));
      mask Help: web(fullfile(path_carnot('help'),'Radiation_on_Inclined_Surface.html'),'-helpbrowser')
      mask TypeOptions sky: isotropic sky | Hay-Davies | Perez 1990
  Select_Weather : Subsystem  mask(Select weather data){v=[6 7]}
      mask prompts: v "vector of index"
      mask help:
      | Selects the indexed weather data from the input weather data vector.
      | Format in weather data vector:
      | 1  timevalue (comment line) format YYYYMMDDHHMM    -
      | 2  zenith angle of sun (at time, not averaged)       degree
      | 3  azimuth angle of sun (0°=south, east negative) degree
      | 4  beam solar radiation on a normal surface         W/m^2
      | 5  diffuse solar radiation on a horizontal surface   W/m^2
      | 6  ambient temperature                                    degree celsius
      | 7  radiation temperature of sky                          degree celsius
      | 8  relative humidity                                           percent
      | 9  precipitation                                                 m/s
      | 10 cloud index (0=no cloud, 1=covered sky)         -
      | 11 station pressure                                           Pa
      | 12 mean wind speed                                         m/s
      | 13 wind direction (north=0° west=270°)             degree
      | 14 incidence angle on surface (0° = vertical)      degree
      | 15 longitudinal incidence angle                       degree
      | 16 transversal incidence angle                        degree
      | 17 direct solar radiation on surface                 W/m²
      | 18 diffuse solar radiation on surface                W/m²
  Tracked_Surface : Subsystem  mask(tracked surface){tracktype=two axis tracking, inc=0, azi=0, rot=0, time=0}
      mask prompts: tracktype "tracking type"; inc "inclination of surface or axis [degrees]"; azi "azimuth of surface or axis (0° = south, -90° = east) [degree]"; rot "rotation of surface or axis [degree]"; time "tracking time [s]"
      mask help: Performs a collector tracking around a given axis. You may specify the time in seconds between two trackings.
      mask Help: web(fullfile(path_carnot('help'),'Tracked_Surface.html'),'-helpbrowser')
      mask TypeOptions tracktype: axis is collector riser | vertical axis | two axis tracking | fixed surface
  WDB2THB : Subsystem  mask(Weather Data Bus to Thermo Hydraulic Bus){dia=0.2}
      mask prompts: dia "diameter [m]"
      mask help: Transfers the incoming weather data to an air flow in the thermo-hydraulic vector THV. All properties are set to ambient conditions (temperature, pressure, humidity).
      mask init:
      | dia = max(dia, 0.001);
      mask Help: web(fullfile(path_carnot('help'),'WDB2THB.html'),'-helpbrowser')
  Weather_Datafile : Subsystem  mask(Weather Datafile){PathName=path_carnot('data'), FileName='DE_TRY2010_04_averageYear.mat', UserParam=off, VariableName=DE_TRY2010_04_averageYear, SampleTime=3600}
      mask prompts: PathName "Selected path"; FileName "File"; UserParam "Edit file and path"; VariableName "Simulink:blkprm_prompts:FromWksData"; SampleTime "Timestep in data"
      mask help:
      | Loads weather data in a variable in the mask workspace and extends it according to the simulation interval. A "From Workspace" block in the subsystem uses this variable. The file must contain data in the weather data format of Carnot (type "help WDB_format" in Command window). A Unit-Delay with the timestep of the data forces the model to a maximum timestep equal to the data timestep. This "Timestep in data" is shown as information in the "Selection" frame.
      | Use of buttons in the "Picking a file" frame:
      | 1) "From selected path" opens a window to chose a data file from the "Selected path" shown in the "Selection" frame.
      | 2) "Carnot public data" opens a window to chose a data file from the public data folder in Carnot. The "Path" is set to the public data folder.
      | 3) "Carnot internal data" opens a window to chose a data file from the internal data folder in Carnot. The "Path" is set to the internal data folder.
      | "File" shows the name of the selected file, "Path" the folder where it is located. You can allow editing "File" and "Path" with the checkbox. Be aware that the buttons in the "Picking a file" frame will anyway overwrite the edited values.
      mask init:
      | [ok,VariableName] = CarnotCallbacks_Data_from_File('LoadData', ...
      |     gcbh, PathName, FileName);
      mask Help: web(fullfile(path_carnot('help'),'WeatherDatafile.html'),'-helpbrowser')
      mask Callback UserParam: ok = CarnotCallbacks_Data_from_File('UserMaskEnable',gcbh);
      mask TypeOptions VariableName: FromWorkspace/VariableName
      mask TypeOptions SampleTime: UnitDelay/SampleTime
      mask DialogControl ParameterGroupVar Prompt: Picking a file
      mask DialogControl Control2 Prompt: From selected path
      mask DialogControl Control2 Callback: ok = CarnotCallbacks_Data_from_File('GetFilename',gcbh, 'selected');
      mask DialogControl Control3 Prompt: Carnot public data
      mask DialogControl Control3 Callback: ok = CarnotCallbacks_Data_from_File('GetFilename',gcbh, 'public');
      mask DialogControl Control4 Prompt: Carnot internal data
      mask DialogControl Control4 Callback: ok = CarnotCallbacks_Data_from_File('GetFilename',gcbh, 'internal');
      mask DialogControl Container3 Prompt: Chosen file
      mask DialogControl VariableName Prompt: Data:
      mask Display: disp(['Weather data file:\n', FileName(1:end-4)])
  Weather_Simple_Model : Subsystem  mask(Weather Simple Model){Ibn=900, Idg=100, tamb=5, deltaTsky=-6, rh=50, precip=10e-3/24/3600           % 10 mm in 24 h, cloud=0.125, p=1013e2, vw=1, wdir=270, lat=50, longi=0, timezone=0, colangle=0, colazi=0, colrot=0}
      mask prompts: Ibn "Maximum beam radiation on normal surface in W/m²"; Idg "Maximum diffuse radiation on horizontal surface in W/m²"; tamb "Ambient temperature in °C"; deltaTsky "Offset for sky temperature in K (usually -6K)"; rh "Relative humidity in %"; precip "Rainfall (precipitation) in m/s"; cloud "Cloud index in (0..1)"; p "Air pressure in Pa"; vw "Wind speed in m/s"; wdir "Wind direction in ° (0° = North, 90° = East)"; lat "Latitude in degree (-90..+90, North postive)"; longi "Longitude in degree (-180..+180, West postive)"; timezone "Longitude of timezone in degree (-180..+180, West postive)"; colangle "Slope of surface (0° = horizontal) [degree]"; colazi "Azimuth of surface (0° = south, -90° = east) [degree]"; colrot "Rotation angle of surface [degree]"
      mask help:
      | Create a simple, mostly constant weather data bus (WDB).
      | The solar radiation corresponds to clear sky conditions.
      mask Help: web(fullfile(path_carnot('help'),'Weather_Simple_Model.html'),'-helpbrowser')
      mask TypeOptions lat: Solar_Position/lati
      mask TypeOptions longi: Solar_Position/longi
      mask TypeOptions timezone: Solar_Position/timezone
      mask TypeOptions colangle: Fixed_Surface/colangle
      mask TypeOptions colazi: Fixed_Surface/colazi
      mask TypeOptions colrot: Fixed_Surface/colrot
      mask DialogControl ParameterTabVar01 Prompt: Weather
      mask DialogControl ParameterTabVar0 Prompt: Geography
      mask DialogControl Container6 Prompt: Surface orientation
      mask Display:
      | plot(0,0,100,100, ...
      |     [10,7,10,20,30,23,25,40,54,56,50,60,70,73,70,60,20,10]*0.8+5, ...
      |     [15,24,34,40,35,42,50,55,50,42,35,40,34,24,15,10,10,15], ...
      |     [70,60,60,70,80,90,90,80,70]*0.7-30,...
      |     [90,80,70,60,60,70,80,90,90],...
      |     [75,75]*0.7-30,[91,97],...
      |     [75,75]*0.7-30,[52,58],...
      |     [58,52]*0.7-30,[75,75],...
      |     [98,91]*0.7-30,[75,75],...
      |     [63,58]*0.7-30,[63,57],...
      |     [92,86]*0.7-30,[92,87],...
      |     [63,58]*0.7-30,[85,92],...
      |     [92,86]*0.7-30,[57,64])
  Weather_from_Workspace : Subsystem  mask(weather from workspace){file=DE_TRY2010_06_averageYear}
      mask prompts: file "Name of variable"
      mask help:
      | Input block for external weather data variables. The variable must be available in the workspace. A "From Workspace" Block is used in the subsystem.
      | A Unit-Delay with the timestep of the weather data forces the model to a maximum timestep equal to the data acquisiton timestep.
      | Remark: Be carefull when using the TRY Data 2010 for Germany. The files are public and can be found in the parameter_set folder of this block. But there are bugs is the solar radiation data.
      mask init:
      | % set variable name in the From Workspace block
      | set_param([gcb '/From_Workspace'], 'VariableName', file);
      | % sample time is timestep of weather data
      | t_sample = evalin('base',eval(['''',eval('file'),'(3,1)'''])) - evalin('base',eval(['''',eval('file'),'(2,1)''']));
      mask Help: web(fullfile(path_carnot('help'),'Weather_from_Workspace.html'),'-helpbrowser')
      mask Display: disp(file)

== system carnot/examples ==
